simulink model "SignalModelL6_aim_p"  (R2017a)
settings: Solver=FixedStepAuto  StartTime=0.0  StopTime=20  FixedStep=0.01  RelTol=1e-3
undefined symbols (not defined in the file): p
settings Model: Creator=roman  LastModifiedBy=roman

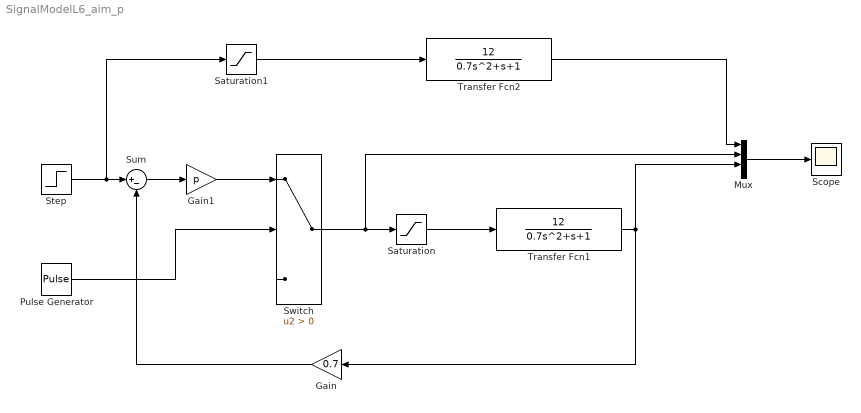
== system SignalModelL6_aim_p ==
  Gain : Gain  Gain=0.7
  Gain1 : Gain  Gain=p
  Mux : Mux
  Pulse Generator : DiscretePulseGenerator  PulseType=Time based  Period=0.1  PulseWidth=50
  Saturation : Saturate  UpperLimit=2000  LowerLimit=-2000
  Saturation1 : Saturate  UpperLimit=2000  LowerLimit=-2000
  Scope : Scope
  Step : Step  Time=0  SampleTime=0
  Sum : Sum  Inputs=|+-
  Switch : Switch  Criteria=u2 > Threshold
  Transfer Fcn1 : TransferFcn  Numerator=[12]  Denominator=[0.7 1 1]
  Transfer Fcn2 : TransferFcn  Numerator=[12]  Denominator=[0.7 1 1]
  wires:
  Saturation1/1 -> Transfer Fcn2/1
  Mux/1 -> Scope/1
  Step/1 -> Sum/1, Saturation1/1
  Transfer Fcn2/1 -> Mux/1
  Saturation/1 -> Transfer Fcn1/1
  Switch/1 -> Mux/2, Saturation/1
  Gain/1 -> Sum/2
  Transfer Fcn1/1 -> Gain/1, Mux/3
  Sum/1 -> Gain1/1
  Pulse Generator/1 -> Switch/2
  Gain1/1 -> Switch/1
